simulink model "sim_part6"  (R2022b)
settings: Solver=VariableStepAuto  StartTime=0.0  StopTime=20.0  RelTol=1e-3
undefined symbols (not defined in the file): K61, K62, matA1, matB1, V6, V7
libraries: cstblocks x12
settings Model: Creator=alon  LastModifiedBy=binya
settings SolverCC: AlgebraicLoopSolver=TrustRegion
settings DebuggingCC: UnconnectedInputMsg=warning  UnconnectedOutputMsg=warning  UnconnectedLineMsg=warning  SFMachineParentedDataDiag=warning
settings ModelReferenceCC: EnableRefExpFcnMdlSchedulingChecks=on

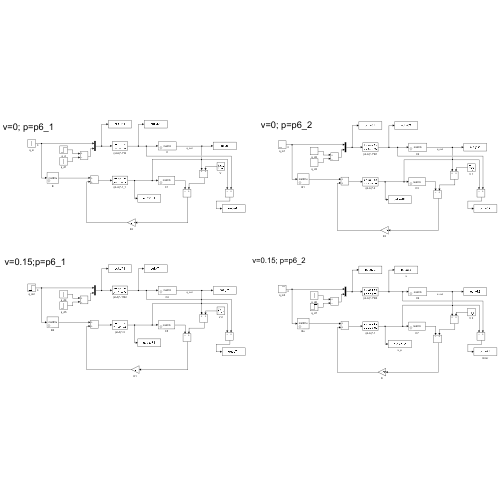
[thumbnail: Simulink's stored preview of the top-level diagram]
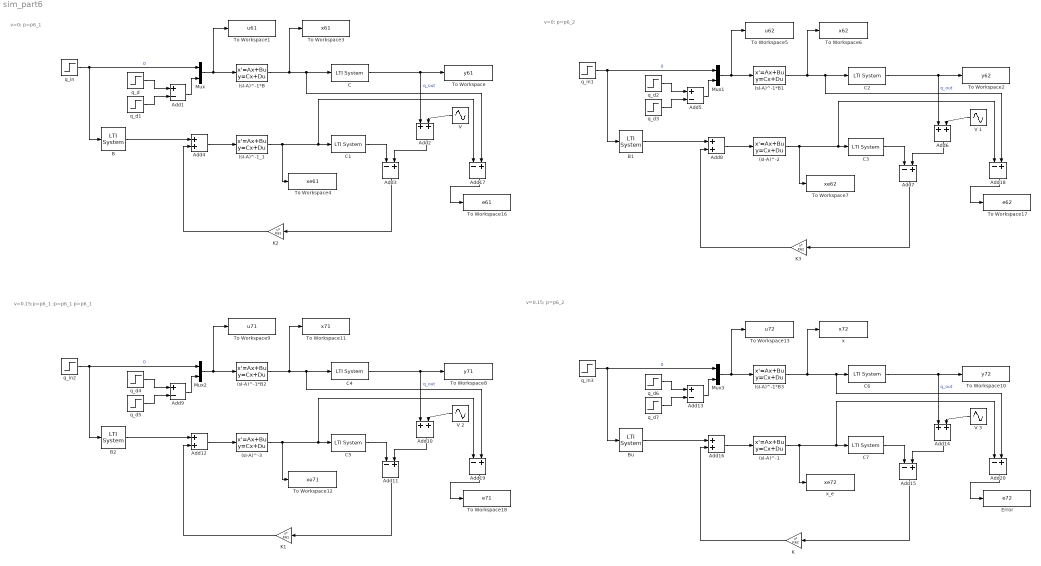
== system sim_part6 ==
  note: v=0; p=p6_1
  note: v=0; p=p6_2
  note: v=0.15;p=p6_1 ;p=p6_1 p=p6_1
  note: v=0.15; p=p6_2
  (sI-A)^-1 : StateSpace  A=matA1  B=eye(3)  C=eye(3)  D=[[0 0 0];[0 0 0];[0 0 0]]  InitialCondition=0
  (sI-A)^-1*B{,1..3} (4 alike) : StateSpace  A=matA1  B=matB1  C=eye(3)  D=[[0 0];[0 0];[0 0]]  InitialCondition=0
  (sI-A)^-1_1 : StateSpace  A=matA1  B=eye(3)  C=eye(3)  D=[[0 0 0];[0 0 0];[0 0 0]]  InitialCondition=0
  (sI-A)^-2 : StateSpace  A=matA1  B=eye(3)  C=eye(3)  D=[[0 0 0];[0 0 0];[0 0 0]]  InitialCondition=0
  (sI-A)^-3 : StateSpace  A=matA1  B=eye(3)  C=eye(3)  D=[[0 0 0];[0 0 0];[0 0 0]]  InitialCondition=0
  Add{1,5,9,13} (4 alike) : Sum  Inputs=+-
  Add{2,4,6,8,10,12,14,16} (8 alike) : Sum
  Add{3,7,11,15,17..20} (8 alike) : Sum  Inputs=-+
  B : cstblocks/LTI System  sys=matB1u  IC=[]
  B1 : cstblocks/LTI System  sys=matB1u  IC=[]
  B2 : cstblocks/LTI System  sys=matB1u  IC=[]
  Bu : cstblocks/LTI System  sys=matB1u  IC=[]
  C{,1..7} (8 alike) : cstblocks/LTI System  sys=matC6  IC=[]
  Error : ToWorkspace  VariableName=e72  SaveFormat=Timeseries  SampleTime=-1
  K : Gain  Gain=K62  Multiplication=Matrix(u*K)
  K1 : Gain  Gain=K61  Multiplication=Matrix(u*K)
  K2 : Gain  Gain=K61  Multiplication=Matrix(u*K)
  K3 : Gain  Gain=K62  Multiplication=Matrix(u*K)
  Mux{,1..3} (4 alike) : Mux  Inputs=2
  To Workspace : ToWorkspace  VariableName=y61  SaveFormat=Timeseries  SampleTime=-1
  To Workspace1 : ToWorkspace  VariableName=u61  SaveFormat=Timeseries  SampleTime=-1
  To Workspace10 : ToWorkspace  VariableName=y72  SaveFormat=Timeseries  SampleTime=-1
  To Workspace11 : ToWorkspace  VariableName=x71  SaveFormat=Timeseries  SampleTime=-1
  To Workspace12 : ToWorkspace  VariableName=xe71  SaveFormat=Timeseries  SampleTime=-1
  To Workspace13 : ToWorkspace  VariableName=u72  SaveFormat=Timeseries  SampleTime=-1
  To Workspace16 : ToWorkspace  VariableName=e61  SaveFormat=Timeseries  SampleTime=-1
  To Workspace17 : ToWorkspace  VariableName=e62  SaveFormat=Timeseries  SampleTime=-1
  To Workspace18 : ToWorkspace  VariableName=e71  SaveFormat=Timeseries  SampleTime=-1
  To Workspace2 : ToWorkspace  VariableName=y62  SaveFormat=Timeseries  SampleTime=-1
  To Workspace3 : ToWorkspace  VariableName=x61  SaveFormat=Timeseries  SampleTime=-1
  To Workspace4 : ToWorkspace  VariableName=xe61  SaveFormat=Timeseries  SampleTime=-1
  To Workspace5 : ToWorkspace  VariableName=u62  SaveFormat=Timeseries  SampleTime=-1
  To Workspace6 : ToWorkspace  VariableName=x62  SaveFormat=Timeseries  SampleTime=-1
  To Workspace7 : ToWorkspace  VariableName=xe62  SaveFormat=Timeseries  SampleTime=-1
  To Workspace8 : ToWorkspace  VariableName=y71  SaveFormat=Timeseries  SampleTime=-1
  To Workspace9 : ToWorkspace  VariableName=u71  SaveFormat=Timeseries  SampleTime=-1
  "V " : Sin  Amplitude=V6  Frequency=10  SampleTime=0
  V 1 : Sin  Amplitude=V6  Frequency=10  SampleTime=0
  V 2 : Sin  Amplitude=V7  Frequency=10  SampleTime=0
  V 3 : Sin  Amplitude=V7  Frequency=10  SampleTime=0
  q_d{,2,4,6} (4 alike) : Step  Time=0  After=12  SampleTime=0
  q_d{1,3,5,7} (4 alike) : Step  Time=2.3  After=12  SampleTime=0
  q_in{,1..3} (4 alike) : Step  Time=0  After=0  SampleTime=0
  x : ToWorkspace  VariableName=x72  SaveFormat=Timeseries  SampleTime=-1
  x_e : ToWorkspace  VariableName=xe72  SaveFormat=Timeseries  SampleTime=-1
  wires:
  Mux/1 -> To Workspace1/1, (sI-A)^-1*B/1
  q_in/1 -> Mux/1, B/1  "0"
  q_d1/1 -> Add1/2
  q_d/1 -> Add1/1
  Add1/1 -> Mux/2
  C/1 -> Add2/1, To Workspace/1  "q_out"
  "V "/1 -> Add2/2
  Add2/1 -> Add3/2
  C1/1 -> Add3/1
  Add3/1 -> K2/1
  K2/1 -> Add4/2
  B/1 -> Add4/1
  Add4/1 -> (sI-A)^-1_1/1
  (sI-A)^-1*B/1 -> Add17/2, C/1, To Workspace3/1
  (sI-A)^-1_1/1 -> Add17/1, C1/1, To Workspace4/1
  V 1/1 -> Add6/2
  C3/1 -> Add7/1
  B1/1 -> Add8/1
  q_in1/1 -> Mux1/1, B1/1  "0"
  Add8/1 -> (sI-A)^-2/1
  q_d3/1 -> Add5/2
  Mux1/1 -> To Workspace5/1, (sI-A)^-1*B1/1
  K3/1 -> Add8/2
  C2/1 -> Add6/1, To Workspace2/1  "q_out"
  Add5/1 -> Mux1/2
  Add6/1 -> Add7/2
  Add7/1 -> K3/1
  q_d2/1 -> Add5/1
  Mux3/1 -> To Workspace13/1, (sI-A)^-1*B3/1
  C6/1 -> Add14/1, To Workspace10/1  "q_out"
  q_d7/1 -> Add13/2
  Add16/1 -> (sI-A)^-1/1
  C7/1 -> Add15/1
  K/1 -> Add16/2
  Add15/1 -> K/1
  V 3/1 -> Add14/2
  q_d6/1 -> Add13/1
  V 2/1 -> Add10/2
  Bu/1 -> Add16/1
  Add14/1 -> Add15/2
  C5/1 -> Add11/1
  Add13/1 -> Mux3/2
  B2/1 -> Add12/1
  q_in2/1 -> Mux2/1, B2/1  "0"
  Add12/1 -> (sI-A)^-3/1
  q_d5/1 -> Add9/2
  Mux2/1 -> To Workspace9/1, (sI-A)^-1*B2/1
  K1/1 -> Add12/2
  C4/1 -> Add10/1, To Workspace8/1  "q_out"
  Add9/1 -> Mux2/2
  Add10/1 -> Add11/2
  Add11/1 -> K1/1
  q_in3/1 -> Mux3/1, Bu/1  "0"
  q_d4/1 -> Add9/1
  Add17/1 -> To Workspace16/1
  (sI-A)^-1*B1/1 -> Add18/2, C2/1, To Workspace6/1
  Add18/1 -> To Workspace17/1
  (sI-A)^-2/1 -> Add18/1, C3/1, To Workspace7/1
  (sI-A)^-1*B2/1 -> Add19/2, C4/1, To Workspace11/1
  Add19/1 -> To Workspace18/1
  (sI-A)^-3/1 -> Add19/1, C5/1, To Workspace12/1
  (sI-A)^-1*B3/1 -> Add20/2, C6/1, x/1
  Add20/1 -> Error/1
  (sI-A)^-1/1 -> Add20/1, C7/1, x_e/1
